simulink model "pv_panel"  (R2026a)
settings: Solver=VariableStepAuto
values from neighbouring files (symbols this model uses):
  I0 = (Isc_stc + Ki*(T - T_stc)) / (exp(Voc_T/Vt) - 1)    [pv_dataset.m]    (also in pv_params.m)
  Iph = (Isc_stc + Ki*(T - T_stc)) * (G / G_stc)    [pv_dataset.m]    (also in pv_params.m = 8.21)
  Rs = 0.221    [pv_dataset.m]    (also in pv_params.m)
  Rsh = 415.405    [pv_dataset.m]    (also in pv_params.m)
  Vt = Ns * n * k * T / q    [pv_dataset.m]    (also in pv_params.m = 1.8036190543)
settings Model: Creator=Mark  LastModifiedBy=Mark

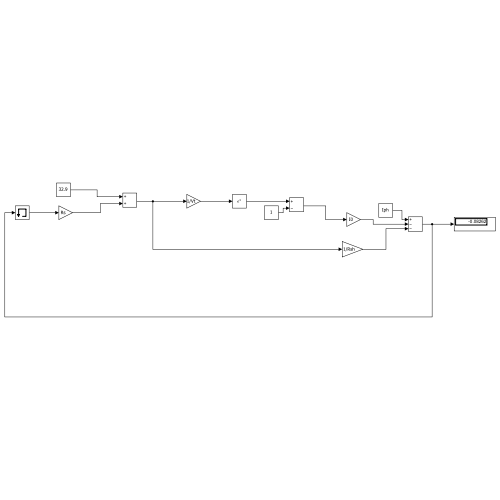
[thumbnail: Simulink's stored preview of the top-level diagram]
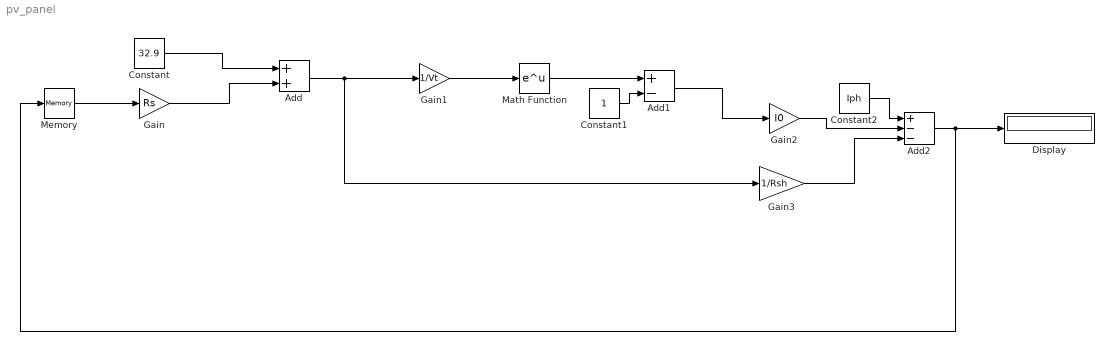
== system pv_panel ==
  Add : Sum
  Add1 : Sum  Inputs=+-
  Add2 : Sum  Inputs=+--
  Constant : Constant  Value=32.9
  Constant1 : Constant
  Constant2 : Constant  Value=Iph
  Display : Display
  Gain : Gain  Gain=Rs
  Gain1 : Gain  Gain=1/Vt
  Gain2 : Gain  Gain=I0
  Gain3 : Gain  Gain=1/Rsh
  Math Function : Math
  Memory : Memory
  wires:
  Constant/1 -> Add/1
  Gain/1 -> Add/2
  Add/1 -> Gain1/1, Gain3/1
  Gain1/1 -> Math Function/1
  Math Function/1 -> Add1/1
  Constant1/1 -> Add1/2
  Add1/1 -> Gain2/1
  Constant2/1 -> Add2/1
  Gain2/1 -> Add2/2
  Gain3/1 -> Add2/3
  Add2/1 -> Memory/1, Display/1
  Memory/1 -> Gain/1
